simulink model "Microgrid_W"  (R2020a)
settings: Solver=ode15s  StartTime=0  StopTime=1440*7  MaxStep=1  RelTol=1e-3
libraries: Microgrid_Library x33, powerlib x1
settings Model: Creator=burmesdani  LastModifiedBy=Daniel
settings SolverCC: ZeroCrossAlgorithm=Adaptive
settings DataIOCC: ReturnWorkspaceOutputs=off
settings DebuggingCC: MaxConsecutiveZCsMsg=none  ArithmeticOperatorsInVariantConditions=warning
settings SFSimCC: SimUseLocalCustomCode=off  CustomCodeUndefinedFunction=UseInterfaceOnly
settings RTWCC: RTWUseLocalCustomCode=off
settings CodeAppCC: StateflowObjectComments=on
settings SimscapeCC: SimscapeNormalizeSystem=off

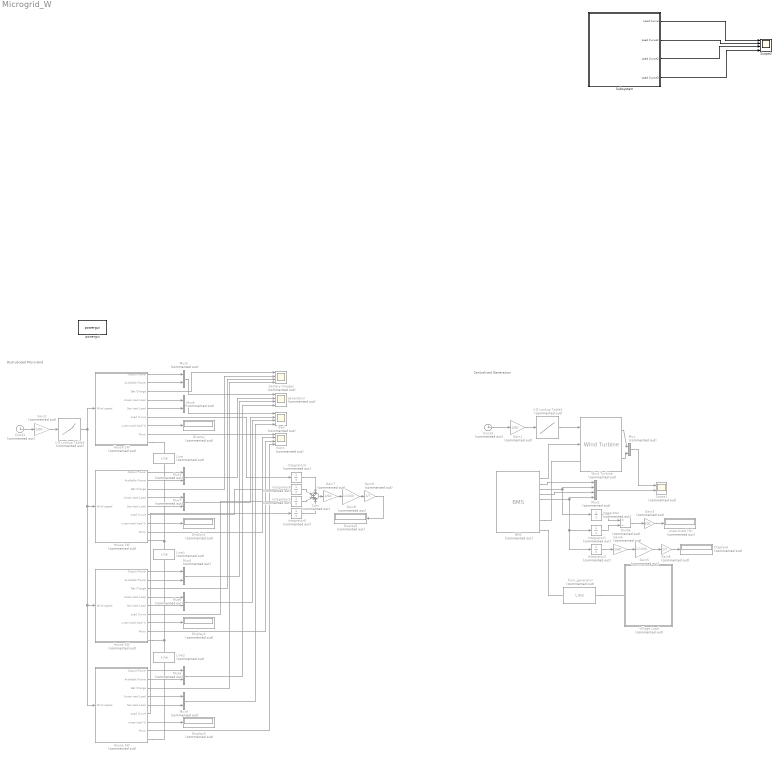
== system Microgrid_W ==
  note: Distrubuted Micro-Grid
  note: Centralised Generation
  1-D Lookup Table1 : Lookup_n-D  Commented=on  NumberOfTableDimensions=1  BreakpointsForDimension1=[ 0 1 2 3 4 5 6 7 8 9 10 11 12 13 14 15 16 17 18 19 20 21 22 23 24 25 26 27 28 29 30 31 32 33 34 35 36 37 38 39 40 41 42 43 44 45 46 47 48 49 50 51 52 53 54 55 56 57 58 59 60 61 62 63 64 65 66 67 68 69 70 71 72 73 74 75 76 77 78 79 80 81 82 83 84 85 86 87 88 89 90 91 92 93 94 95 96 97 98 99 100 101 102 103 104 105 106 107 108 109 110 111 112 113 114 115 116 117 118 119 120 121 122 123 124 125 126 127 128 129 130 131 132 133 134 135 136 137 138 139 140 141 142 143 144 145 146 147 148 149 150 151 152 153 154 155 156 157 158 159 160 161 162 163 164 165 166 167 ]  Table=|  InternalRulePriority=Speed  RndMeth=Simplest  InputSameDT=on
      | [7.2
      | 6.6
      | 7.7
      | 4.6
      | 6.1
      | 5.6
      | 6.1
      | 6.6
      | 5.6
      | 5.6
      | 5.6
      | 5.1
      | 9.2
      | 7.7
      | 6.6
      | 6.1
      | 6.6
      | 6.1
      | 5.6
      | 6.1
      | 4.1
      | 2.5
      | 1.5
      | 3
      | 3.6
      | 4.1
      | 3
      | 3
      | 2
      | 1
      | 1.5
      | 1.5
      | 3
      | 4.6
      | 4.6
      | 5.1
      | 5.1
      | 7.7
      | 8.7
      | 6.6
      | 7.2
      | 6.1
      | 6.6
      | 6.1
      | 5.6
      | 6.1
      | 7.7
      | 8.7
      | 9.2
      | 8.7
      | 8.2
      | 7.7
      | 8.7
      | 9.2
      | 10.8
      | 9.2
      | 8.7
      | 9.2
      | 9.2
      | 12.3
      | 9.7
      | 8.2
      | 5.1
      | 7.2
      | 8.2
      | 7.2
      | 8.2
      | 6.6
      | 7.2
      | 5.6
      | 5.6
      | 5.6
      | 4.1
      | 5.1
      | 5.6
      | 5.1
      | 3
      | 4.1
      | 2.5
      | 1.5
      | 0.5
      | 1
      | 0
      | 6.6
      | 9.2
      | 11.3
      | 11.8
      | 8.2
      | 7.2
      | 6.1
      | 6.1
      | 4.6
      | 4.6
      | 4.1
      | 4.1
      | 3.6
      | 3
      | 2
      | 2
      | 2
      | 2
      | 2.5
      | 2
      | 2
      | 1.5
      | 1
      | 0
      | 2.5
      | 2.5
      | 3
      | 3.6
      | 3.6
      | 4.1
      | 4.6
      | 3.6
      | 2.5
      | 2.5
      | 2.5
      | 1.5
      | 5.1
      | 4.6
      | 5.1
      | 7.2
      | 6.6
      | 8.2
      | 5.6
      | 4.6
      | 2.5
      | 1
      | 1
      | 5.1
      | 10.3
      | 11.3
      | 11.3
      | 11.8
      | 10.8
      | 9.7
      | 9.2
      | 9.2
      | 8.2
      | 8.2
      | 7.7
      | 6.6
      | 7.2
      | 3.6
      | 5.6
      | 2
      | 3
      | 2.5
      | 2
      | 2.5
      | 2
      | 2
      | 2
      | 2
      | 2.5
      | 3
      | 3
      | 5.6
      | 7.7
      | 9.2
      | 10.3
      | 11.8
      | 15.4
      | 15.4
      | 15.4
      | 14.9
      | 12.8]
  1-D Lookup Table2 : Lookup_n-D  Commented=on  NumberOfTableDimensions=1  BreakpointsForDimension1=[ 0 1 2 3 4 5 6 7 8 9 10 11 12 13 14 15 16 17 18 19 20 21 22 23 24 25 26 27 28 29 30 31 32 33 34 35 36 37 38 39 40 41 42 43 44 45 46 47 48 49 50 51 52 53 54 55 56 57 58 59 60 61 62 63 64 65 66 67 68 69 70 71 72 73 74 75 76 77 78 79 80 81 82 83 84 85 86 87 88 89 90 91 92 93 94 95 96 97 98 99 100 101 102 103 104 105 106 107 108 109 110 111 112 113 114 115 116 117 118 119 120 121 122 123 124 125 126 127 128 129 130 131 132 133 134 135 136 137 138 139 140 141 142 143 144 145 146 147 148 149 150 151 152 153 154 155 156 157 158 159 160 161 162 163 164 165 166 167 ]  Table=|  InternalRulePriority=Speed  RndMeth=Simplest  InputSameDT=on
      | [7.2
      | 6.6
      | 7.7
      | 4.6
      | 6.1
      | 5.6
      | 6.1
      | 6.6
      | 5.6
      | 5.6
      | 5.6
      | 5.1
      | 9.2
      | 7.7
      | 6.6
      | 6.1
      | 6.6
      | 6.1
      | 5.6
      | 6.1
      | 4.1
      | 2.5
      | 1.5
      | 3
      | 3.6
      | 4.1
      | 3
      | 3
      | 2
      | 1
      | 1.5
      | 1.5
      | 3
      | 4.6
      | 4.6
      | 5.1
      | 5.1
      | 7.7
      | 8.7
      | 6.6
      | 7.2
      | 6.1
      | 6.6
      | 6.1
      | 5.6
      | 6.1
      | 7.7
      | 8.7
      | 9.2
      | 8.7
      | 8.2
      | 7.7
      | 8.7
      | 9.2
      | 10.8
      | 9.2
      | 8.7
      | 9.2
      | 9.2
      | 12.3
      | 9.7
      | 8.2
      | 5.1
      | 7.2
      | 8.2
      | 7.2
      | 8.2
      | 6.6
      | 7.2
      | 5.6
      | 5.6
      | 5.6
      | 4.1
      | 5.1
      | 5.6
      | 5.1
      | 3
      | 4.1
      | 2.5
      | 1.5
      | 0.5
      | 1
      | 0
      | 6.6
      | 9.2
      | 11.3
      | 11.8
      | 8.2
      | 7.2
      | 6.1
      | 6.1
      | 4.6
      | 4.6
      | 4.1
      | 4.1
      | 3.6
      | 3
      | 2
      | 2
      | 2
      | 2
      | 2.5
      | 2
      | 2
      | 1.5
      | 1
      | 0
      | 2.5
      | 2.5
      | 3
      | 3.6
      | 3.6
      | 4.1
      | 4.6
      | 3.6
      | 2.5
      | 2.5
      | 2.5
      | 1.5
      | 5.1
      | 4.6
      | 5.1
      | 7.2
      | 6.6
      | 8.2
      | 5.6
      | 4.6
      | 2.5
      | 1
      | 1
      | 5.1
      | 10.3
      | 11.3
      | 11.3
      | 11.8
      | 10.8
      | 9.7
      | 9.2
      | 9.2
      | 8.2
      | 8.2
      | 7.7
      | 6.6
      | 7.2
      | 3.6
      | 5.6
      | 2
      | 3
      | 2.5
      | 2
      | 2.5
      | 2
      | 2
      | 2
      | 2
      | 2.5
      | 3
      | 3
      | 5.6
      | 7.7
      | 9.2
      | 10.3
      | 11.8
      | 15.4
      | 15.4
      | 15.4
      | 14.9
      | 12.8]
  BMS : Microgrid_Library/BMS  Commented=on  v=240  c=425
  Clock1 : Clock  Commented=on
  Clock2 : Clock  Commented=on
  Display{,1..5} (6 alike) : Display  Commented=on
  Divide : Product  Commented=on  Inputs=*/
  Gain{1..2,4,7} (4 alike) : Gain  Commented=on  Gain=1/60
  Gain3 : Gain  Commented=on  Gain=100
  Gain5 : Gain  Commented=on  Gain=1/1000
  Gain6 : Gain  Commented=on  Gain=1/7
  Gain8 : Gain  Commented=on  Gain=1/1000
  Gain9 : Gain  Commented=on  Gain=1/7
  House 2W : Subsystem  Commented=on
  House 3W : Subsystem  Commented=on
  House 4W : Subsystem  Commented=on
  House 5W : Subsystem  Commented=on
  Integrator{,1..6} (7 alike) : Integrator  Commented=on
  Line : Microgrid_Library/Line  Commented=on  l=60
  Line1 : Microgrid_Library/Line  Commented=on  l=58
  Line2 : Microgrid_Library/Line  Commented=on  l=47
  Mux{,2..9} (9 alike) : Mux  Commented=on  Inputs=2
  Mux1 : Mux  Commented=on
  Scope1 : Scope  Commented=on  NumInputPorts=2
  Scope2 : Scope  NumInputPorts=4
  Subsystem : Subsystem
  Sum : Sum  Commented=on  Inputs=++++
  Village Load : Subsystem  Commented=on
  Wind Turbine : Microgrid_Library/Wind Turbine  Commented=on  V=240  W=10900
  battery charges : Scope  Commented=on  NumInputPorts=4
  from_generator : Microgrid_Library/Line  Commented=on  l=161
  generation : Scope  Commented=on  NumInputPorts=4
  load : Scope  Commented=on  NumInputPorts=4
  micro : Scope  Commented=on  NumInputPorts=4
  powergui : powerlib/powergui  Priority=1  SimulationMode=Continuous  SampleTime=50e-6  frequency=60  Iterations=50  frequencyindice=0  Pbase=100e6  ErrMax=1e-4  UnitsV=kV  UnitsW=MW  buscounter=0  FunctionMessages=off  echomessages=off  EnableUseOfTLC=off  CurrentSourceSwitches=off  DisableSnubberDevices=off  DisableRonSwitches=off  DisableVfSwitches=off  DisplayEquations=off  AutomaticDiscreteSolvers=off  SolverType=Tustin/Backward Euler (TBE)  Interpol=off  ExternalGateDelay=off  methode=off  Ts=100  x0status=blocks  SPID=on  SwTol=0  HookPort=off  NonlinearTolerance=1e-4  nMaxIteration=100  ContinueOnMaxIteration=off  RestoreLinks=warning  ResistiveCurrentMeasurement=off  Frange=[0:2:500]  Ylog=off  Xlog=on  ShowGrid=off  save=off  variable=ZData  structure=0  ZoomFFT=off  StartTime=0.0  cycles=1  DisplayStyle=1  fundamental=60  FreqAxis=off  MaxFrequency=1000  frequencyindicesteady=1  RmsSteady=1  display=off
  unserviced (%) : Display  Commented=on
  wires:
  House 5W/7(unserviced %) -> Display3/1
  House 2W/7(unserviced load %) -> Display/1
  Clock1/1 -> Gain2/1
  House 4W/7(unserviced load %) -> Display2/1
  House 3W/7(unserviced load %) -> Display1/1
  1-D Lookup Table2/1 -> House 5W/1(Wind speed), House 4W/1(Wind speed), House 3W/1(Wind speed), House 2W/1(Wind speed)
  Gain2/1 -> 1-D Lookup Table2/1
  BMS/5 -> Mux1/3
  Clock2/1 -> Gain1/1
  Divide/1 -> Gain3/1
  Gain5/1 -> Gain6/1
  Integrator2/1 -> Gain4/1
  Wind Turbine/1 -> Mux/1
  BMS/4 -> Mux1/2, Integrator/1
  BMS/6 -> Mux1/4, Integrator2/1, Integrator1/1
  1-D Lookup Table1/1 -> Wind Turbine/1
  BMS/2 -> Wind Turbine/2
  Integrator1/1 -> Divide/2
  Gain6/1 -> Display4/1
  BMS/3 -> Mux1/1
  Gain4/1 -> Gain5/1
  Mux/1 -> Scope1/1
  Wind Turbine/2 -> Mux/2
  Gain1/1 -> 1-D Lookup Table1/1
  Integrator/1 -> Divide/1
  Mux1/1 -> Scope1/2
  Gain3/1 -> unserviced (%)/1
  House 2W/3(Bat Charge) -> battery charges/1
  House 3W/3(Bat Charge) -> battery charges/2
  House 4W/3(Bat Charge) -> battery charges/3
  House 5W/3(Bat Charge) -> battery charges/4
  House 2W/1(Output Power) -> Mux2/1
  House 2W/2(Available Power) -> Mux2/2
  House 3W/1(Output Power) -> Mux3/1
  House 3W/2(Available Power) -> Mux3/2
  House 4W/1(Output Power) -> Mux4/1
  House 4W/2(Available Power) -> Mux4/2
  House 5W/1(Output Power) -> Mux5/1
  House 5W/2(Available Power) -> Mux5/2
  Mux2/1 -> generation/1
  Mux3/1 -> generation/2
  Mux4/1 -> generation/3
  Mux5/1 -> generation/4
  House 2W/4(Unserviced Load) -> Mux6/1
  House 2W/5(Serviced Load) -> Mux6/2
  House 3W/4(Unserviced Load) -> Mux7/1
  House 3W/5(Serviced Load) -> Mux7/2
  House 4W/4(Unserviced Load) -> Mux8/1
  House 4W/5(Serviced Load) -> Mux8/2
  House 5W/4(Unserviced Load) -> Mux9/1
  House 5W/5(Serviced Load) -> Mux9/2
  Mux6/1 -> load/1
  Mux7/1 -> load/2
  Mux8/1 -> load/3
  Mux9/1 -> load/4
  House 2W/8(Micro) -> micro/1
  House 3W/8(Micro) -> micro/2
  House 4W/8(Micro) -> micro/3
  House 5W/8(Micro) -> micro/4
  Gain9/1 -> Display5/1
  Gain8/1 -> Gain9/1
  Gain7/1 -> Gain8/1
  House 2W/6(Load Curve) -> Integrator3/1
  House 3W/6(Load Curve) -> Integrator4/1
  House 4W/6(Load Curve) -> Integrator5/1
  House 5W/6(Load Curve) -> Integrator6/1
  Integrator3/1 -> Sum/1
  Integrator4/1 -> Sum/2
  Integrator5/1 -> Sum/3
  Integrator6/1 -> Sum/4
  Sum/1 -> Gain7/1
  Subsystem/1(Load Curve) -> Scope2/1
  Subsystem/2(Load Curve1) -> Scope2/2
  Subsystem/3(Load Curve2) -> Scope2/3
  Subsystem/4(Load Curve3) -> Scope2/4
  connections:
  House 2W/RConn1 -- Line/LConn1
  Line/RConn1 -- House 3W/RConn1 -- Line1/LConn1
  House 5W/RConn1 -- Line2/RConn1
  House 4W/RConn1 -- Line1/RConn1 -- Line2/LConn1
  BMS/RConn4 -- from_generator/LConn1
  BMS/RConn2 -- Wind Turbine/LConn1
  from_generator/RConn1 -- Village Load/LConn1

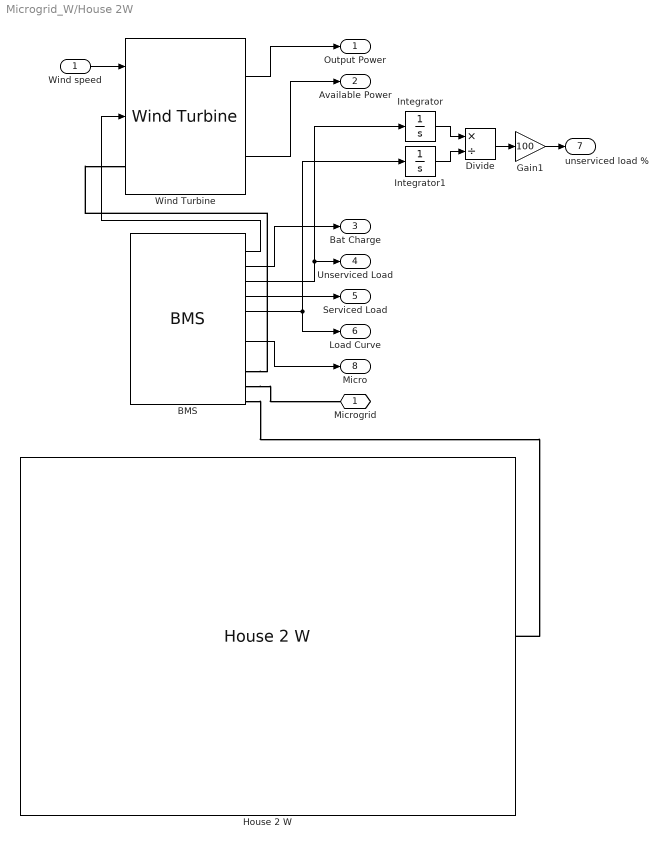
== system Microgrid_W/House 2W ==
  Wind speed : Inport
  BMS : Microgrid_Library/BMS  v=240  c=80
  Divide : Product  Inputs=*/
  Gain1 : Gain  Gain=100
  House 2 W : Microgrid_Library/House 2 W  V=240  t=60  K_L1_W=40  K_L1_On_1=63000  K_L1_Off_1=72600  K_L1_On_2=0  K_L1_Off_2=0  Dishwasher_W=1200  Dishwasher_On=72000  Fridge_W=150  T_Initial=1.9  T_Low=1  T_High=2.4  Jug_W=1500  Jug_On_1=25200  Jug_On_2=64200  Jug_On_3=0  Toaster_W=900  Toaster_On_1=23400  Toaster_On_2=27120  N_Elements=4  Oven_On_1=63600  Oven_Off_1=67200  Shower_On_a=21720  Shower_L_a=240  Shower_On_b=23640  Shower_L_b=300  Shower_On_c=0  Shower_L_c=0  K_L3_W=60  K_L3_On_1=21480  K_L3_Off_1=22140  K_L3_On_2=23580  K_L3_Off_2=24780  HW_W=2000  M=177  D=0.488  L=1.72  Ti=7  Ta=20  T_Low_WH=58  T_High_WH=61  Clock_1_W=5  Lamp_1_W=18  L1_On_1=79740  L1_Off_1=83040  L1_On_2=0  L1_Off_2=0  K_L4_W=24  K_L4_On_1=21000  K_L4_Off_1=27360  Clock_2_W=6  Lamp_2_W=24  L2_On_1=26820  L2_Off_1=29160  L2_On_2=73800  L2_Off_2=76800  K_L5_W=40  K_L5_On_1=28800  K_L5_Off_1=30240  K_L5_On_2=72300  K_L5_Off_2=83880  Phone_C_1_W=3  Phone_C_1_On_a=0  Phone_C_1_Off_a=35700  Phone_C_1_On_b=76800  Phone_C_1_Off_b=86400  Phone_C_2_W=7  Phone_C_2_On_a=0  Phone_C_2_Off_a=35760  Phone_C_2_On_b=76800  Phone_C_2_Off_b=86400  Phone_C_3_W=5  Phone_C_3_On_a=0  Phone_C_3_Off_a=35700  Phone_C_3_On_b=77040  Phone_C_3_Off_b=86400  Laptop_C_1_W=55  Laptop_C_1_On_a=76800  Laptop_C_1_Off_a=86400  Laptop_C_2_W=65  Laptop_C_2_On_a=0  Laptop_C_2_Off_a=28500  Laptop_C_2_On_b=77160  Laptop_C_2_Off_b=86400  Lamp_3_W=60  L3_On_1=21600  L3_Off_1=27000  L3_On_2=62760  L3_Off_2=83220  K_L6_W=60  K_L6_On_1=68400  K_L6_Off_1=70200  Heater_W=1800  Heater_On_1=62040  Heater_Off_1=68640  Stereo_W=100  Stereo_On_1=42480  Stereo_Off_1=58200  TV_W=500  TV_On_1=21900  TV_Off_1=26580  TV_On_2=63000  TV_Off_2=73200
  Integrator : Integrator
  Integrator1 : Integrator
  Wind Turbine : Microgrid_Library/Wind Turbine  V=240  W=2000
  Microgrid : PMIOPort  Side=Right
  Output Power : Outport
  Available Power : Outport  Port=2
  Bat Charge : Outport  Port=3
  Unserviced Load : Outport  Port=4
  Serviced Load : Outport  Port=5
  Load Curve : Outport  Port=6
  unserviced load % : Outport  Port=7
  Micro : Outport  Port=8
  wires:
  Wind Turbine/2 -> Available Power/1
  Wind Turbine/1 -> Output Power/1
  BMS/2 -> Wind Turbine/2
  Wind speed/1 -> Wind Turbine/1
  BMS/3 -> Bat Charge/1
  BMS/5 -> Serviced Load/1
  BMS/8 -> Micro/1
  BMS/4 -> Integrator/1, Unserviced Load/1
  Integrator1/1 -> Divide/2
  BMS/6 -> Load Curve/1, Integrator1/1
  Gain1/1 -> unserviced load %/1
  Integrator/1 -> Divide/1
  Divide/1 -> Gain1/1
  connections:
  BMS/RConn2 -- Wind Turbine/LConn1
  BMS/RConn4 -- House 2 W/LConn1
  BMS/RConn3 -- Microgrid/RConn1

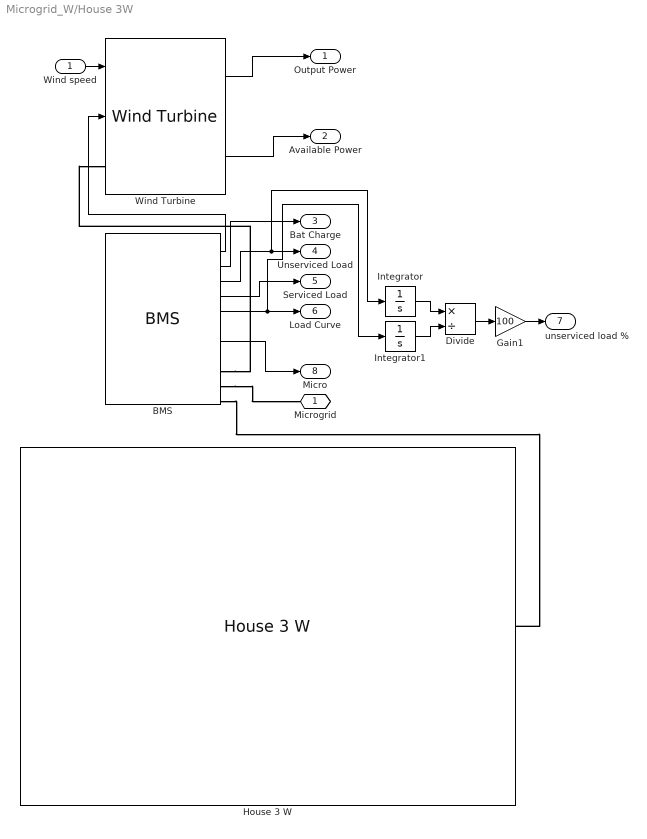
== system Microgrid_W/House 3W ==
  Wind speed : Inport
  BMS : Microgrid_Library/BMS  v=240  c=95
  Divide : Product  Inputs=*/
  Gain1 : Gain  Gain=100
  House 3 W : Microgrid_Library/House 3 W  V=240  t=60  K_L1_W=24  K_L1_On_1=21600  K_L1_Off_1=26580  K_L1_On_2=63000  K_L1_Off_2=68400  K_L2_W=60  K_L2_On_1=63000  K_L2_Off_1=68400  Fridge_W=200  T_Initial=1.5  T_Low=1.5  T_High=2.65  Jug_W=2000  Jug_On_1=21720  Jug_On_2=43560  Jug_On_3=73800  Toaster_W=1200  Toaster_On_1=25260  Toaster_On_2=28920  N_Elements=1  Oven_On_1=58680  Oven_Off_1=68760  Shower_On_a=70440  Shower_L_a=360  Shower_On_b=76740  Shower_L_b=180  Shower_On_c=81000  Shower_L_c=180  K_L3_W=80  K_L3_On_1=70200  K_L3_Off_1=70800  K_L3_On_2=76320  K_L3_Off_2=81300  HW_W=3000  M=250  D=0.58  L=1.56  Ti=7  Ta=20  T_Low_WH=59  T_High_WH=61  Clock_1_W=6  Lamp_1_W=18  L1_On_1=71400  L1_Off_1=81120  L1_On_2=0  L1_Off_2=0  K_L4_W=60  K_L4_On_1=69600  K_L4_Off_1=71400  Clock_2_W=4  Lamp_2_W=24  L2_On_1=84120  L2_Off_1=86880  L2_On_2=0  L2_Off_2=0  K_L5_W=40  K_L5_On_1=25320  K_L5_Off_1=28980  K_L5_On_2=81000  K_L5_Off_2=84180  Phone_C_1_W=7  Phone_C_1_On_a=0  Phone_C_1_Off_a=27300  Phone_C_1_On_b=79200  Phone_C_1_Off_b=86400  Phone_C_2_W=6  Phone_C_2_On_a=0  Phone_C_2_Off_a=27300  Phone_C_2_On_b=79200  Phone_C_2_Off_b=86400  Phone_C_3_W=5  Phone_C_3_On_a=0  Phone_C_3_Off_a=0  Phone_C_3_On_b=0  Phone_C_3_Off_b=0  Laptop_C_1_W=1  Laptop_C_1_On_a=0  Laptop_C_1_Off_a=0  Laptop_C_2_W=45  Laptop_C_2_On_a=0  Laptop_C_2_Off_a=6000  Laptop_C_2_On_b=66600  Laptop_C_2_Off_b=86400  Lamp_3_W=40  L3_On_1=24900  L3_Off_1=30600  L3_On_2=72000  L3_Off_2=81000  K_L6_W=60  K_L6_On_1=68760  K_L6_Off_1=71520  Heater_W=1500  Heater_On_1=64800  Heater_Off_1=78000  Stereo_W=1  Stereo_On_1=0  Stereo_Off_1=0  TV_W=150  TV_On_1=25200  TV_Off_1=28800  TV_On_2=72240  TV_Off_2=81000
  Integrator : Integrator
  Integrator1 : Integrator
  Wind Turbine : Microgrid_Library/Wind Turbine  V=240  W=2600
  Microgrid : PMIOPort  Side=Right
  Output Power : Outport
  Available Power : Outport  Port=2
  Bat Charge : Outport  Port=3
  Unserviced Load : Outport  Port=4
  Serviced Load : Outport  Port=5
  Load Curve : Outport  Port=6
  unserviced load % : Outport  Port=7
  Micro : Outport  Port=8
  wires:
  Wind speed/1 -> Wind Turbine/1
  Wind Turbine/1 -> Output Power/1
  BMS/4 -> Integrator/1, Unserviced Load/1
  BMS/6 -> Integrator1/1, Load Curve/1
  BMS/2 -> Wind Turbine/2
  BMS/3 -> Bat Charge/1
  Wind Turbine/2 -> Available Power/1
  BMS/5 -> Serviced Load/1
  BMS/8 -> Micro/1
  Gain1/1 -> unserviced load %/1
  Integrator/1 -> Divide/1
  Integrator1/1 -> Divide/2
  Divide/1 -> Gain1/1
  connections:
  BMS/RConn4 -- House 3 W/LConn1
  BMS/RConn2 -- Wind Turbine/LConn1
  BMS/RConn3 -- Microgrid/RConn1

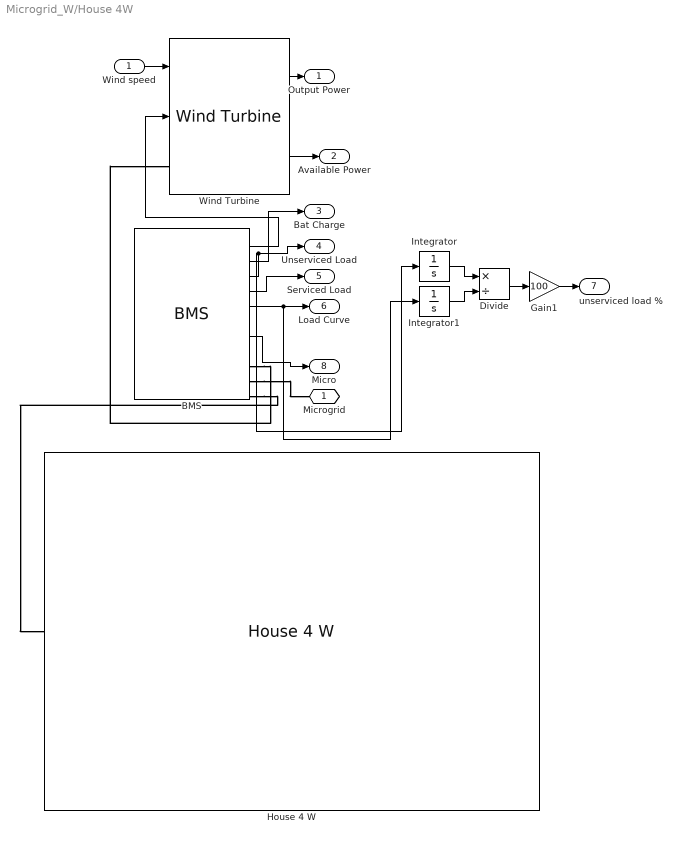
== system Microgrid_W/House 4W ==
  Wind speed : Inport
  BMS : Microgrid_Library/BMS  v=240  c=85
  Divide : Product  Inputs=*/
  Gain1 : Gain  Gain=100
  House 4 W : Microgrid_Library/House 4 W  V=240  t=60  K_L1_W=60  K_L1_On_1=69180  K_L1_Off_1=70200  K_L1_On_2=0  K_L1_Off_2=0  K_L2_W=1  K_L2_On_1=0  K_L2_Off_1=0  Fridge_W=150  T_Initial=1  T_Low=1  T_High=3.6  Jug_W=1800  Jug_On_1=23760  Jug_On_2=79800  Jug_On_3=0  Toaster_W=1000  Toaster_On_1=21600  Toaster_On_2=0  N_Elements=2  Oven_On_1=69240  Oven_Off_1=70140  Shower_On_a=20040  Shower_L_a=180  Shower_On_b=0  Shower_L_b=0  Shower_On_c=0  Shower_L_c=0  K_L3_W=40  K_L3_On_1=19800  K_L3_Off_1=20400  K_L3_On_2=0  K_L3_Off_2=0  HW_W=2000  M=88  D=0.488  L=0.955  Ti=7  Ta=20  T_Low_WH=55  T_High_WH=59.5  Clock_1_W=0  Lamp_1_W=1  L1_On_1=0  L1_Off_1=0  L1_On_2=0  L1_Off_2=0  K_L4_W=1  K_L4_On_1=0  K_L4_Off_1=0  Clock_2_W=4  Lamp_2_W=40  L2_On_1=19680  L2_Off_1=21600  L2_On_2=82800  L2_Off_2=84600  K_L5_W=1  K_L5_On_1=0  K_L5_Off_1=0  K_L5_On_2=0  K_L5_Off_2=0  Phone_C_1_W=5  Phone_C_1_On_a=0  Phone_C_1_Off_a=27300  Phone_C_1_On_b=79200  Phone_C_1_Off_b=86400  Phone_C_2_W=0  Phone_C_2_On_a=0  Phone_C_2_Off_a=0  Phone_C_2_On_b=0  Phone_C_2_Off_b=0  Phone_C_3_W=0  Phone_C_3_On_a=0  Phone_C_3_Off_a=0  Phone_C_3_On_b=0  Phone_C_3_Off_b=0  Laptop_C_1_W=35  Laptop_C_1_On_a=63900  Laptop_C_1_Off_a=75600  Laptop_C_2_W=65  Laptop_C_2_On_a=0  Laptop_C_2_Off_a=21600  Laptop_C_2_On_b=66600  Laptop_C_2_Off_b=86400  Lamp_3_W=18  L3_On_1=66000  L3_Off_1=82800  L3_On_2=0  L3_Off_2=0  K_L6_W=40  K_L6_On_1=63000  K_L6_Off_1=66000  Heater_W=2000  Heater_On_1=65100  Heater_Off_1=82200  Stereo_W=100  Stereo_On_1=68640  Stereo_Off_1=70740  TV_W=300  TV_On_1=70800  TV_Off_1=82800  TV_On_2=0  TV_Off_2=0
  Integrator : Integrator
  Integrator1 : Integrator
  Wind Turbine : Microgrid_Library/Wind Turbine  V=240  W=1800
  Microgrid : PMIOPort  Side=Right
  Output Power : Outport
  Available Power : Outport  Port=2
  Bat Charge : Outport  Port=3
  Unserviced Load : Outport  Port=4
  Serviced Load : Outport  Port=5
  Load Curve : Outport  Port=6
  unserviced load % : Outport  Port=7
  Micro : Outport  Port=8
  wires:
  BMS/2 -> Wind Turbine/2
  BMS/3 -> Bat Charge/1
  BMS/4 -> Unserviced Load/1, Integrator/1
  Wind Turbine/2 -> Available Power/1
  Wind speed/1 -> Wind Turbine/1
  Wind Turbine/1 -> Output Power/1
  BMS/6 -> Integrator1/1, Load Curve/1
  BMS/5 -> Serviced Load/1
  BMS/8 -> Micro/1
  Gain1/1 -> unserviced load %/1
  Integrator/1 -> Divide/1
  Divide/1 -> Gain1/1
  Integrator1/1 -> Divide/2
  connections:
  BMS/RConn4 -- House 4 W/LConn1
  BMS/RConn2 -- Wind Turbine/LConn1
  BMS/RConn3 -- Microgrid/RConn1

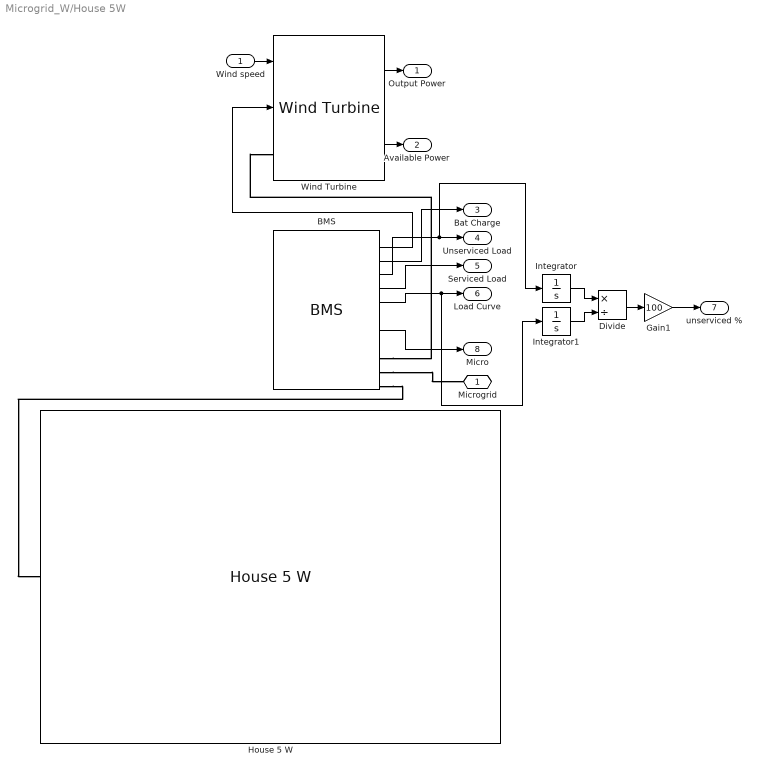
== system Microgrid_W/House 5W ==
  Wind speed : Inport
  BMS : Microgrid_Library/BMS  v=240  c=165
  Divide : Product  Inputs=*/
  Gain1 : Gain  Gain=100
  House 5 W : Microgrid_Library/House 5 W  V=240  t=60  K_L1_W=18  K_L1_On_1=23220  K_L1_Off_1=27120  K_L1_On_2=74160  K_L1_Off_2=82020  Dishwasher_W=1200  Dishwasher_On=36420  Fridge_W=150  T_Initial=1.35  T_Low=1.2  T_High=3.1  Jug_W=1500  Jug_On_1=25620  Jug_On_2=0  Jug_On_3=0  Toaster_W=1100  Toaster_On_1=30600  Toaster_On_2=0  N_Elements=4  Oven_On_1=65040  Oven_Off_1=69900  Shower_On_a=29100  Shower_L_a=240  Shower_On_b=39000  Shower_L_b=300  Shower_On_c=0  Shower_L_c=0  K_L3_W=18  K_L3_On_1=28800  K_L3_Off_1=29400  K_L3_On_2=38700  K_L3_Off_2=39120  HW_W=2000  M=135  D=0.488  L=1.35  Ti=7  Ta=20  T_Low_WH=56  T_High_WH=58  Clock_1_W=3  Lamp_1_W=18  L1_On_1=70560  L1_Off_1=82920  L1_On_2=0  L1_Off_2=0  K_L4_W=40  K_L4_On_1=65400  K_L4_Off_1=76200  Clock_2_W=5  Lamp_2_W=18  L2_On_1=26640  L2_Off_1=29520  L2_On_2=66000  L2_Off_2=79560  K_L5_W=60  K_L5_On_1=77100  K_L5_Off_1=79560  K_L5_On_2=0  K_L5_Off_2=0  Phone_C_1_W=5  Phone_C_1_On_a=0  Phone_C_1_Off_a=8760  Phone_C_1_On_b=77100  Phone_C_1_Off_b=86400  Phone_C_2_W=6  Phone_C_2_On_a=0  Phone_C_2_Off_a=21600  Phone_C_2_On_b=77100  Phone_C_2_Off_b=86400  Phone_C_3_W=5  Phone_C_3_On_a=0  Phone_C_3_Off_a=14820  Phone_C_3_On_b=77100  Phone_C_3_Off_b=86400  Laptop_C_1_W=65  Laptop_C_1_On_a=34200  Laptop_C_1_Off_a=52200  Laptop_C_2_W=65  Laptop_C_2_On_a=72780  Laptop_C_2_Off_a=77100  Laptop_C_2_On_b=0  Laptop_C_2_Off_b=0  Lamp_3_W=24  L3_On_1=25200  L3_Off_1=27000  L3_On_2=20040  L3_Off_2=84000  K_L6_W=100  K_L6_On_1=70200  K_L6_Off_1=73800  Heater_W=2000  Heater_On_1=29160  Heater_Off_1=76140  Stereo_W=50  Stereo_On_1=43560  Stereo_Off_1=45480  TV_W=200  TV_On_1=39900  TV_Off_1=52200  TV_On_2=69600  TV_Off_2=77100
  Integrator : Integrator
  Integrator1 : Integrator
  Wind Turbine : Microgrid_Library/Wind Turbine  V=240  W=4500
  Microgrid : PMIOPort  Side=Right
  Output Power : Outport
  Available Power : Outport  Port=2
  Bat Charge : Outport  Port=3
  Unserviced Load : Outport  Port=4
  Serviced Load : Outport  Port=5
  Load Curve : Outport  Port=6
  unserviced % : Outport  Port=7
  Micro : Outport  Port=8
  wires:
  BMS/5 -> Serviced Load/1
  Wind Turbine/2 -> Available Power/1
  BMS/2 -> Wind Turbine/2
  Wind speed/1 -> Wind Turbine/1
  Wind Turbine/1 -> Output Power/1
  BMS/4 -> Integrator/1, Unserviced Load/1
  BMS/6 -> Integrator1/1, Load Curve/1
  BMS/3 -> Bat Charge/1
  BMS/8 -> Micro/1
  Integrator1/1 -> Divide/2
  Divide/1 -> Gain1/1
  Integrator/1 -> Divide/1
  Gain1/1 -> unserviced %/1
  connections:
  BMS/RConn3 -- Microgrid/RConn1
  BMS/RConn4 -- House 5 W/LConn1
  BMS/RConn2 -- Wind Turbine/LConn1

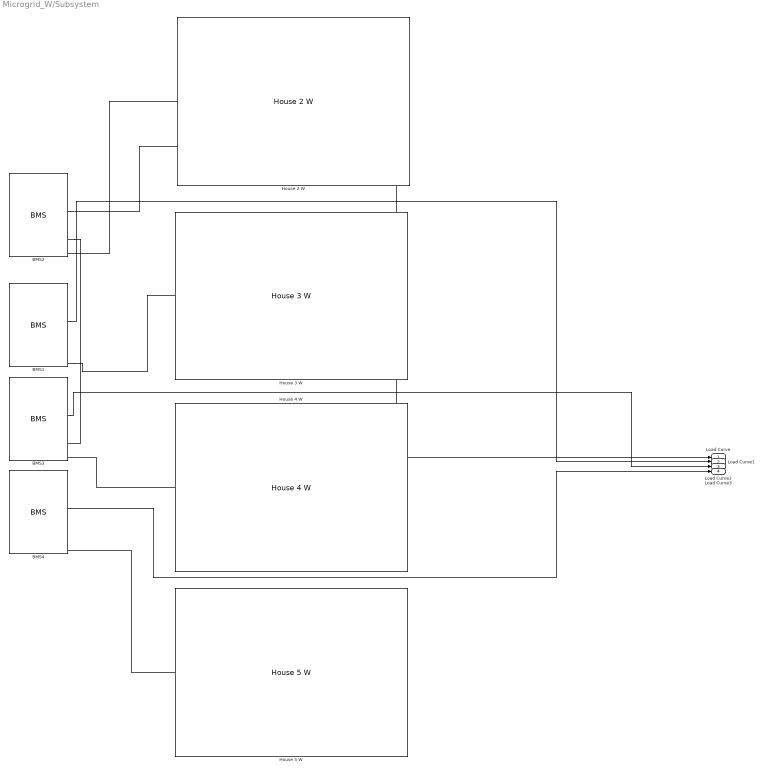
== system Microgrid_W/Subsystem ==
  BMS{1..4} (4 alike) : Microgrid_Library/BMS  v=240  c=425
  House 2 W : Microgrid_Library/House 2 W  V=240  t=60  K_L1_W=40  K_L1_On_1=63000  K_L1_Off_1=72600  K_L1_On_2=0  K_L1_Off_2=0  Dishwasher_W=1200  Dishwasher_On=72000  Fridge_W=150  T_Initial=1.9  T_Low=1  T_High=2.4  Jug_W=1500  Jug_On_1=25200  Jug_On_2=64200  Jug_On_3=0  Toaster_W=900  Toaster_On_1=23400  Toaster_On_2=27120  N_Elements=4  Oven_On_1=63600  Oven_Off_1=67200  Shower_On_a=21720  Shower_L_a=240  Shower_On_b=23640  Shower_L_b=300  Shower_On_c=0  Shower_L_c=0  K_L3_W=60  K_L3_On_1=21480  K_L3_Off_1=22140  K_L3_On_2=23580  K_L3_Off_2=24780  HW_W=2000  M=177  D=0.488  L=1.72  Ti=7  Ta=20  T_Low_WH=58  T_High_WH=61  Clock_1_W=5  Lamp_1_W=18  L1_On_1=79740  L1_Off_1=83040  L1_On_2=0  L1_Off_2=0  K_L4_W=24  K_L4_On_1=21000  K_L4_Off_1=27360  Clock_2_W=6  Lamp_2_W=24  L2_On_1=26820  L2_Off_1=29160  L2_On_2=73800  L2_Off_2=76800  K_L5_W=40  K_L5_On_1=28800  K_L5_Off_1=30240  K_L5_On_2=72300  K_L5_Off_2=83880  Phone_C_1_W=3  Phone_C_1_On_a=0  Phone_C_1_Off_a=35700  Phone_C_1_On_b=76800  Phone_C_1_Off_b=86400  Phone_C_2_W=7  Phone_C_2_On_a=0  Phone_C_2_Off_a=35760  Phone_C_2_On_b=76800  Phone_C_2_Off_b=86400  Phone_C_3_W=5  Phone_C_3_On_a=0  Phone_C_3_Off_a=35700  Phone_C_3_On_b=77040  Phone_C_3_Off_b=86400  Laptop_C_1_W=55  Laptop_C_1_On_a=76800  Laptop_C_1_Off_a=86400  Laptop_C_2_W=65  Laptop_C_2_On_a=0  Laptop_C_2_Off_a=28500  Laptop_C_2_On_b=77160  Laptop_C_2_Off_b=86400  Lamp_3_W=60  L3_On_1=21600  L3_Off_1=27000  L3_On_2=62760  L3_Off_2=83220  K_L6_W=60  K_L6_On_1=68400  K_L6_Off_1=70200  Heater_W=1800  Heater_On_1=62040  Heater_Off_1=68640  Stereo_W=100  Stereo_On_1=42480  Stereo_Off_1=58200  TV_W=500  TV_On_1=21900  TV_Off_1=26580  TV_On_2=63000  TV_Off_2=73200
  House 3 W : Microgrid_Library/House 3 W  V=240  t=60  K_L1_W=24  K_L1_On_1=21600  K_L1_Off_1=26580  K_L1_On_2=63000  K_L1_Off_2=68400  K_L2_W=60  K_L2_On_1=63000  K_L2_Off_1=68400  Fridge_W=200  T_Initial=1.5  T_Low=1.5  T_High=2.65  Jug_W=2000  Jug_On_1=21720  Jug_On_2=43560  Jug_On_3=73800  Toaster_W=1200  Toaster_On_1=25260  Toaster_On_2=28920  N_Elements=1  Oven_On_1=58680  Oven_Off_1=68760  Shower_On_a=70440  Shower_L_a=360  Shower_On_b=76740  Shower_L_b=180  Shower_On_c=81000  Shower_L_c=180  K_L3_W=80  K_L3_On_1=70200  K_L3_Off_1=70800  K_L3_On_2=76320  K_L3_Off_2=81300  HW_W=3000  M=250  D=0.58  L=1.56  Ti=7  Ta=20  T_Low_WH=59  T_High_WH=61  Clock_1_W=6  Lamp_1_W=18  L1_On_1=71400  L1_Off_1=81120  L1_On_2=0  L1_Off_2=0  K_L4_W=60  K_L4_On_1=69600  K_L4_Off_1=71400  Clock_2_W=4  Lamp_2_W=24  L2_On_1=84120  L2_Off_1=86880  L2_On_2=0  L2_Off_2=0  K_L5_W=40  K_L5_On_1=25320  K_L5_Off_1=28980  K_L5_On_2=81000  K_L5_Off_2=84180  Phone_C_1_W=7  Phone_C_1_On_a=0  Phone_C_1_Off_a=27300  Phone_C_1_On_b=79200  Phone_C_1_Off_b=86400  Phone_C_2_W=6  Phone_C_2_On_a=0  Phone_C_2_Off_a=27300  Phone_C_2_On_b=79200  Phone_C_2_Off_b=86400  Phone_C_3_W=5  Phone_C_3_On_a=0  Phone_C_3_Off_a=0  Phone_C_3_On_b=0  Phone_C_3_Off_b=0  Laptop_C_1_W=1  Laptop_C_1_On_a=0  Laptop_C_1_Off_a=0  Laptop_C_2_W=45  Laptop_C_2_On_a=0  Laptop_C_2_Off_a=6000  Laptop_C_2_On_b=66600  Laptop_C_2_Off_b=86400  Lamp_3_W=40  L3_On_1=24900  L3_Off_1=30600  L3_On_2=72000  L3_Off_2=81000  K_L6_W=60  K_L6_On_1=68760  K_L6_Off_1=71520  Heater_W=1500  Heater_On_1=64800  Heater_Off_1=78000  Stereo_W=1  Stereo_On_1=0  Stereo_Off_1=0  TV_W=150  TV_On_1=25200  TV_Off_1=28800  TV_On_2=72240  TV_Off_2=81000
  House 4 W : Microgrid_Library/House 4 W  V=240  t=60  K_L1_W=60  K_L1_On_1=69180  K_L1_Off_1=70200  K_L1_On_2=0  K_L1_Off_2=0  K_L2_W=1  K_L2_On_1=0  K_L2_Off_1=0  Fridge_W=150  T_Initial=1  T_Low=1  T_High=3.6  Jug_W=1800  Jug_On_1=23760  Jug_On_2=79800  Jug_On_3=0  Toaster_W=1000  Toaster_On_1=21600  Toaster_On_2=0  N_Elements=2  Oven_On_1=69240  Oven_Off_1=70140  Shower_On_a=20040  Shower_L_a=180  Shower_On_b=0  Shower_L_b=0  Shower_On_c=0  Shower_L_c=0  K_L3_W=40  K_L3_On_1=19800  K_L3_Off_1=20400  K_L3_On_2=0  K_L3_Off_2=0  HW_W=2000  M=88  D=0.488  L=0.955  Ti=7  Ta=20  T_Low_WH=55  T_High_WH=59.5  Clock_1_W=0  Lamp_1_W=1  L1_On_1=0  L1_Off_1=0  L1_On_2=0  L1_Off_2=0  K_L4_W=1  K_L4_On_1=0  K_L4_Off_1=0  Clock_2_W=4  Lamp_2_W=40  L2_On_1=19680  L2_Off_1=21600  L2_On_2=82800  L2_Off_2=84600  K_L5_W=1  K_L5_On_1=0  K_L5_Off_1=0  K_L5_On_2=0  K_L5_Off_2=0  Phone_C_1_W=5  Phone_C_1_On_a=0  Phone_C_1_Off_a=27300  Phone_C_1_On_b=79200  Phone_C_1_Off_b=86400  Phone_C_2_W=0  Phone_C_2_On_a=0  Phone_C_2_Off_a=0  Phone_C_2_On_b=0  Phone_C_2_Off_b=0  Phone_C_3_W=0  Phone_C_3_On_a=0  Phone_C_3_Off_a=0  Phone_C_3_On_b=0  Phone_C_3_Off_b=0  Laptop_C_1_W=35  Laptop_C_1_On_a=63900  Laptop_C_1_Off_a=75600  Laptop_C_2_W=65  Laptop_C_2_On_a=0  Laptop_C_2_Off_a=21600  Laptop_C_2_On_b=66600  Laptop_C_2_Off_b=86400  Lamp_3_W=18  L3_On_1=66000  L3_Off_1=82800  L3_On_2=0  L3_Off_2=0  K_L6_W=40  K_L6_On_1=63000  K_L6_Off_1=66000  Heater_W=2000  Heater_On_1=65100  Heater_Off_1=82200  Stereo_W=100  Stereo_On_1=68640  Stereo_Off_1=70740  TV_W=300  TV_On_1=70800  TV_Off_1=82800  TV_On_2=0  TV_Off_2=0
  House 5 W : Microgrid_Library/House 5 W  V=240  t=60  K_L1_W=18  K_L1_On_1=23220  K_L1_Off_1=27120  K_L1_On_2=74160  K_L1_Off_2=82020  Dishwasher_W=1200  Dishwasher_On=36420  Fridge_W=150  T_Initial=1.35  T_Low=1.2  T_High=3.1  Jug_W=1500  Jug_On_1=25620  Jug_On_2=0  Jug_On_3=0  Toaster_W=1100  Toaster_On_1=30600  Toaster_On_2=0  N_Elements=4  Oven_On_1=65040  Oven_Off_1=69900  Shower_On_a=29100  Shower_L_a=240  Shower_On_b=39000  Shower_L_b=300  Shower_On_c=0  Shower_L_c=0  K_L3_W=18  K_L3_On_1=28800  K_L3_Off_1=29400  K_L3_On_2=38700  K_L3_Off_2=39120  HW_W=2000  M=135  D=0.488  L=1.35  Ti=7  Ta=20  T_Low_WH=56  T_High_WH=58  Clock_1_W=3  Lamp_1_W=18  L1_On_1=70560  L1_Off_1=82920  L1_On_2=0  L1_Off_2=0  K_L4_W=40  K_L4_On_1=65400  K_L4_Off_1=76200  Clock_2_W=5  Lamp_2_W=18  L2_On_1=26640  L2_Off_1=29520  L2_On_2=66000  L2_Off_2=79560  K_L5_W=60  K_L5_On_1=77100  K_L5_Off_1=79560  K_L5_On_2=0  K_L5_Off_2=0  Phone_C_1_W=5  Phone_C_1_On_a=0  Phone_C_1_Off_a=8760  Phone_C_1_On_b=77100  Phone_C_1_Off_b=86400  Phone_C_2_W=6  Phone_C_2_On_a=0  Phone_C_2_Off_a=21600  Phone_C_2_On_b=77100  Phone_C_2_Off_b=86400  Phone_C_3_W=5  Phone_C_3_On_a=0  Phone_C_3_Off_a=14820  Phone_C_3_On_b=77100  Phone_C_3_Off_b=86400  Laptop_C_1_W=65  Laptop_C_1_On_a=34200  Laptop_C_1_Off_a=52200  Laptop_C_2_W=65  Laptop_C_2_On_a=72780  Laptop_C_2_Off_a=77100  Laptop_C_2_On_b=0  Laptop_C_2_Off_b=0  Lamp_3_W=24  L3_On_1=25200  L3_Off_1=27000  L3_On_2=20040  L3_Off_2=84000  K_L6_W=100  K_L6_On_1=70200  K_L6_Off_1=73800  Heater_W=2000  Heater_On_1=29160  Heater_Off_1=76140  Stereo_W=50  Stereo_On_1=43560  Stereo_Off_1=45480  TV_W=200  TV_On_1=39900  TV_Off_1=52200  TV_On_2=69600  TV_Off_2=77100
  Load Curve : Outport
  Load Curve1 : Outport  Port=2
  Load Curve2 : Outport  Port=3
  Load Curve3 : Outport  Port=4
  wires:
  BMS2/6 -> Load Curve/1
  BMS1/6 -> Load Curve1/1
  BMS3/6 -> Load Curve2/1
  BMS4/6 -> Load Curve3/1
  connections:
  BMS2/RConn2 -- BMS3/RConn2
  House 4 W/LConn1 -- BMS3/RConn4
  House 5 W/LConn1 -- BMS4/RConn4
  BMS1/RConn4 -- House 3 W/LConn1
  House 2 W/LConn1 -- BMS2/RConn4

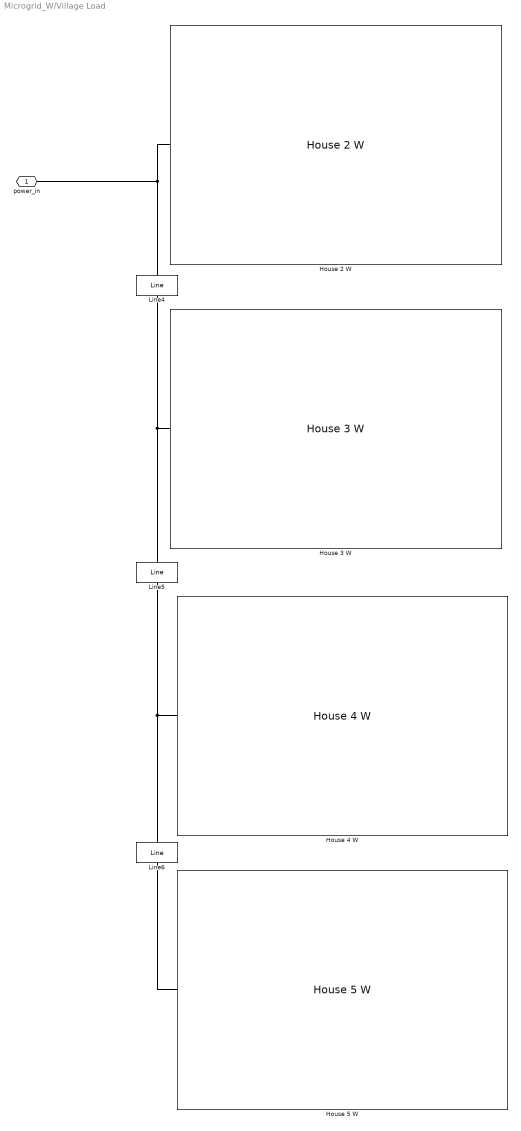
== system Microgrid_W/Village Load ==
  House 2 W : Microgrid_Library/House 2 W  V=240  t=60  K_L1_W=40  K_L1_On_1=63000  K_L1_Off_1=72600  K_L1_On_2=0  K_L1_Off_2=0  Dishwasher_W=1200  Dishwasher_On=72000  Fridge_W=150  T_Initial=1.9  T_Low=1  T_High=2.4  Jug_W=1500  Jug_On_1=25200  Jug_On_2=64200  Jug_On_3=0  Toaster_W=900  Toaster_On_1=23400  Toaster_On_2=27120  N_Elements=4  Oven_On_1=63600  Oven_Off_1=67200  Shower_On_a=21720  Shower_L_a=240  Shower_On_b=23640  Shower_L_b=300  Shower_On_c=0  Shower_L_c=0  K_L3_W=60  K_L3_On_1=21480  K_L3_Off_1=22140  K_L3_On_2=23580  K_L3_Off_2=24780  HW_W=2000  M=177  D=0.488  L=1.72  Ti=7  Ta=20  T_Low_WH=58  T_High_WH=61  Clock_1_W=5  Lamp_1_W=18  L1_On_1=79740  L1_Off_1=83040  L1_On_2=0  L1_Off_2=0  K_L4_W=24  K_L4_On_1=21000  K_L4_Off_1=27360  Clock_2_W=6  Lamp_2_W=24  L2_On_1=26820  L2_Off_1=29160  L2_On_2=73800  L2_Off_2=76800  K_L5_W=40  K_L5_On_1=28800  K_L5_Off_1=30240  K_L5_On_2=72300  K_L5_Off_2=83880  Phone_C_1_W=3  Phone_C_1_On_a=0  Phone_C_1_Off_a=35700  Phone_C_1_On_b=76800  Phone_C_1_Off_b=86400  Phone_C_2_W=7  Phone_C_2_On_a=0  Phone_C_2_Off_a=35760  Phone_C_2_On_b=76800  Phone_C_2_Off_b=86400  Phone_C_3_W=5  Phone_C_3_On_a=0  Phone_C_3_Off_a=35700  Phone_C_3_On_b=77040  Phone_C_3_Off_b=86400  Laptop_C_1_W=55  Laptop_C_1_On_a=76800  Laptop_C_1_Off_a=86400  Laptop_C_2_W=65  Laptop_C_2_On_a=0  Laptop_C_2_Off_a=28500  Laptop_C_2_On_b=77160  Laptop_C_2_Off_b=86400  Lamp_3_W=60  L3_On_1=21600  L3_Off_1=27000  L3_On_2=62760  L3_Off_2=83220  K_L6_W=60  K_L6_On_1=68400  K_L6_Off_1=70200  Heater_W=1800  Heater_On_1=62040  Heater_Off_1=68640  Stereo_W=100  Stereo_On_1=42480  Stereo_Off_1=58200  TV_W=500  TV_On_1=21900  TV_Off_1=26580  TV_On_2=63000  TV_Off_2=73200
  House 3 W : Microgrid_Library/House 3 W  V=240  t=60  K_L1_W=24  K_L1_On_1=21600  K_L1_Off_1=26580  K_L1_On_2=63000  K_L1_Off_2=68400  K_L2_W=60  K_L2_On_1=63000  K_L2_Off_1=68400  Fridge_W=200  T_Initial=1.5  T_Low=1.5  T_High=2.65  Jug_W=2000  Jug_On_1=21720  Jug_On_2=43560  Jug_On_3=73800  Toaster_W=1200  Toaster_On_1=25260  Toaster_On_2=28920  N_Elements=1  Oven_On_1=58680  Oven_Off_1=68760  Shower_On_a=70440  Shower_L_a=360  Shower_On_b=76740  Shower_L_b=180  Shower_On_c=81000  Shower_L_c=180  K_L3_W=80  K_L3_On_1=70200  K_L3_Off_1=70800  K_L3_On_2=76320  K_L3_Off_2=81300  HW_W=3000  M=250  D=0.58  L=1.56  Ti=7  Ta=20  T_Low_WH=59  T_High_WH=61  Clock_1_W=6  Lamp_1_W=18  L1_On_1=71400  L1_Off_1=81120  L1_On_2=0  L1_Off_2=0  K_L4_W=60  K_L4_On_1=69600  K_L4_Off_1=71400  Clock_2_W=4  Lamp_2_W=24  L2_On_1=84120  L2_Off_1=86880  L2_On_2=0  L2_Off_2=0  K_L5_W=40  K_L5_On_1=25320  K_L5_Off_1=28980  K_L5_On_2=81000  K_L5_Off_2=84180  Phone_C_1_W=7  Phone_C_1_On_a=0  Phone_C_1_Off_a=27300  Phone_C_1_On_b=79200  Phone_C_1_Off_b=86400  Phone_C_2_W=6  Phone_C_2_On_a=0  Phone_C_2_Off_a=27300  Phone_C_2_On_b=79200  Phone_C_2_Off_b=86400  Phone_C_3_W=5  Phone_C_3_On_a=0  Phone_C_3_Off_a=0  Phone_C_3_On_b=0  Phone_C_3_Off_b=0  Laptop_C_1_W=1  Laptop_C_1_On_a=0  Laptop_C_1_Off_a=0  Laptop_C_2_W=45  Laptop_C_2_On_a=0  Laptop_C_2_Off_a=6000  Laptop_C_2_On_b=66600  Laptop_C_2_Off_b=86400  Lamp_3_W=40  L3_On_1=24900  L3_Off_1=30600  L3_On_2=72000  L3_Off_2=81000  K_L6_W=60  K_L6_On_1=68760  K_L6_Off_1=71520  Heater_W=1500  Heater_On_1=64800  Heater_Off_1=78000  Stereo_W=1  Stereo_On_1=0  Stereo_Off_1=0  TV_W=150  TV_On_1=25200  TV_Off_1=28800  TV_On_2=72240  TV_Off_2=81000
  House 4 W : Microgrid_Library/House 4 W  V=240  t=60  K_L1_W=60  K_L1_On_1=69180  K_L1_Off_1=70200  K_L1_On_2=0  K_L1_Off_2=0  K_L2_W=1  K_L2_On_1=0  K_L2_Off_1=0  Fridge_W=150  T_Initial=1  T_Low=1  T_High=3.6  Jug_W=1800  Jug_On_1=23760  Jug_On_2=79800  Jug_On_3=0  Toaster_W=1000  Toaster_On_1=21600  Toaster_On_2=0  N_Elements=2  Oven_On_1=69240  Oven_Off_1=70140  Shower_On_a=20040  Shower_L_a=180  Shower_On_b=0  Shower_L_b=0  Shower_On_c=0  Shower_L_c=0  K_L3_W=40  K_L3_On_1=19800  K_L3_Off_1=20400  K_L3_On_2=0  K_L3_Off_2=0  HW_W=2000  M=88  D=0.488  L=0.955  Ti=7  Ta=20  T_Low_WH=55  T_High_WH=59.5  Clock_1_W=0  Lamp_1_W=1  L1_On_1=0  L1_Off_1=0  L1_On_2=0  L1_Off_2=0  K_L4_W=1  K_L4_On_1=0  K_L4_Off_1=0  Clock_2_W=4  Lamp_2_W=40  L2_On_1=19680  L2_Off_1=21600  L2_On_2=82800  L2_Off_2=84600  K_L5_W=1  K_L5_On_1=0  K_L5_Off_1=0  K_L5_On_2=0  K_L5_Off_2=0  Phone_C_1_W=5  Phone_C_1_On_a=0  Phone_C_1_Off_a=27300  Phone_C_1_On_b=79200  Phone_C_1_Off_b=86400  Phone_C_2_W=0  Phone_C_2_On_a=0  Phone_C_2_Off_a=0  Phone_C_2_On_b=0  Phone_C_2_Off_b=0  Phone_C_3_W=0  Phone_C_3_On_a=0  Phone_C_3_Off_a=0  Phone_C_3_On_b=0  Phone_C_3_Off_b=0  Laptop_C_1_W=35  Laptop_C_1_On_a=63900  Laptop_C_1_Off_a=75600  Laptop_C_2_W=65  Laptop_C_2_On_a=0  Laptop_C_2_Off_a=21600  Laptop_C_2_On_b=66600  Laptop_C_2_Off_b=86400  Lamp_3_W=18  L3_On_1=66000  L3_Off_1=82800  L3_On_2=0  L3_Off_2=0  K_L6_W=40  K_L6_On_1=63000  K_L6_Off_1=66000  Heater_W=2000  Heater_On_1=65100  Heater_Off_1=82200  Stereo_W=100  Stereo_On_1=68640  Stereo_Off_1=70740  TV_W=300  TV_On_1=70800  TV_Off_1=82800  TV_On_2=0  TV_Off_2=0
  House 5 W : Microgrid_Library/House 5 W  V=240  t=60  K_L1_W=18  K_L1_On_1=23220  K_L1_Off_1=27120  K_L1_On_2=74160  K_L1_Off_2=82020  Dishwasher_W=1200  Dishwasher_On=36420  Fridge_W=150  T_Initial=1.35  T_Low=1.2  T_High=3.1  Jug_W=1500  Jug_On_1=25620  Jug_On_2=0  Jug_On_3=0  Toaster_W=1100  Toaster_On_1=30600  Toaster_On_2=0  N_Elements=4  Oven_On_1=65040  Oven_Off_1=69900  Shower_On_a=29100  Shower_L_a=240  Shower_On_b=39000  Shower_L_b=300  Shower_On_c=0  Shower_L_c=0  K_L3_W=18  K_L3_On_1=28800  K_L3_Off_1=29400  K_L3_On_2=38700  K_L3_Off_2=39120  HW_W=2000  M=135  D=0.488  L=1.35  Ti=7  Ta=20  T_Low_WH=56  T_High_WH=58  Clock_1_W=3  Lamp_1_W=18  L1_On_1=70560  L1_Off_1=82920  L1_On_2=0  L1_Off_2=0  K_L4_W=40  K_L4_On_1=65400  K_L4_Off_1=76200  Clock_2_W=5  Lamp_2_W=18  L2_On_1=26640  L2_Off_1=29520  L2_On_2=66000  L2_Off_2=79560  K_L5_W=60  K_L5_On_1=77100  K_L5_Off_1=79560  K_L5_On_2=0  K_L5_Off_2=0  Phone_C_1_W=5  Phone_C_1_On_a=0  Phone_C_1_Off_a=8760  Phone_C_1_On_b=77100  Phone_C_1_Off_b=86400  Phone_C_2_W=6  Phone_C_2_On_a=0  Phone_C_2_Off_a=21600  Phone_C_2_On_b=77100  Phone_C_2_Off_b=86400  Phone_C_3_W=5  Phone_C_3_On_a=0  Phone_C_3_Off_a=14820  Phone_C_3_On_b=77100  Phone_C_3_Off_b=86400  Laptop_C_1_W=65  Laptop_C_1_On_a=34200  Laptop_C_1_Off_a=52200  Laptop_C_2_W=65  Laptop_C_2_On_a=72780  Laptop_C_2_Off_a=77100  Laptop_C_2_On_b=0  Laptop_C_2_Off_b=0  Lamp_3_W=24  L3_On_1=25200  L3_Off_1=27000  L3_On_2=20040  L3_Off_2=84000  K_L6_W=100  K_L6_On_1=70200  K_L6_Off_1=73800  Heater_W=2000  Heater_On_1=29160  Heater_Off_1=76140  Stereo_W=50  Stereo_On_1=43560  Stereo_Off_1=45480  TV_W=200  TV_On_1=39900  TV_Off_1=52200  TV_On_2=69600  TV_Off_2=77100
  Line4 : Microgrid_Library/Line  l=60
  Line5 : Microgrid_Library/Line  l=58
  Line6 : Microgrid_Library/Line  l=47
  power_in : PMIOPort  Side=Left
  connections:
  power_in/RConn1 -- Line4/LConn1 -- House 2 W/LConn1
  Line6/RConn1 -- House 5 W/LConn1
  Line4/RConn1 -- Line5/LConn1 -- House 3 W/LConn1
  Line6/LConn1 -- Line5/RConn1 -- House 4 W/LConn1
